simulink model "Lab4_6_StudentVersion"  (R2025a)
settings: Solver=VariableStepAuto  StartTime=0.0  StopTime=30  FixedStep=5e-5  MaxStep=1e-4  RelTol=1e-6
values from neighbouring files (symbols this model uses):
  Ke1 = 10    [ParametersLAb4_6_StudentVersion.m]
  Ke2 = 10    [ParametersLAb4_6_StudentVersion.m]
  Ki = 4.5e-4    (= 0.00045)    [ParametersLAb4_6_StudentVersion.m]
  Ksi = 1    [ParametersLAb4_6_StudentVersion.m]
  m1 = delta_w/P1_rated    (= 0.00333333333333)    [ParametersLAb4_6_StudentVersion.m]
  m2 = delta_w/P2_rated    (= 0.0025)    [ParametersLAb4_6_StudentVersion.m]
  n1 = delta_V/Q1_rated    (= 0.000666666666667)    [ParametersLAb4_6_StudentVersion.m]
  n2 = delta_V/Q2_rated    (= 0.00133333333333)    [ParametersLAb4_6_StudentVersion.m]
  P1_rated = 3000    [ParametersLAb4_6_StudentVersion.m]
  P2_rated = 4000    [ParametersLAb4_6_StudentVersion.m]
  Q1_rated = 1500    [ParametersLAb4_6_StudentVersion.m]
  Q2_rated = 1500/2    (= 750)    [ParametersLAb4_6_StudentVersion.m]
  Rf = 0.1    [ParametersLAb4_6_StudentVersion.m]
  T32 = sqrt(2/3)*[   1      0 ... (first row only)    [ParametersLAb4_6_StudentVersion.m]
  Tf = 0.1    [ParametersLAb4_6_StudentVersion.m]
  V1_rated = 110    [ParametersLAb4_6_StudentVersion.m]
  V2_rated = 110    [ParametersLAb4_6_StudentVersion.m]
  w1_rated = 2*pi*f1_rated    (= 376.991118431)    [ParametersLAb4_6_StudentVersion.m]
  w2_rated = 2*pi*f2_rated    (= 376.991118431)    [ParametersLAb4_6_StudentVersion.m]
  wne = 500    [ParametersLAb4_6_StudentVersion.m]
libraries: fl_lib x33, nesl_utility x31, ee_lib x22
(part 2 of 2)

== system Lab4_6_StudentVersion/Subsystem8 ==
  PS-Simulink Converter : nesl_utility/PS-Simulink Converter  PhysicalDomain=network_engine_domain  SubClassName=ps_output  LeftPortType=input  RightPortType=output  PseudoPeriodic=off  Frequencies=[]  VectorFormat=inherit  Unit=inherit  AffineConversion=off
  Voltage Sensor : fl_lib/Electrical/Electrical Sensors/Voltage Sensor
  + : PMIOPort  Side=Right
  - : PMIOPort  Port=2  Side=Right
  V : Outport
  wires:
  PS-Simulink Converter/1 -> V/1
  connections:
  Voltage Sensor/RConn2 -- -/RConn1
  PS-Simulink Converter/LConn1 -- Voltage Sensor/RConn1
  Voltage Sensor/LConn1 -- +/RConn1

== system Lab4_6_StudentVersion/Subsystem9 ==
  PS-Simulink Converter : nesl_utility/PS-Simulink Converter  PhysicalDomain=network_engine_domain  SubClassName=ps_output  LeftPortType=input  RightPortType=output  PseudoPeriodic=off  Frequencies=[]  VectorFormat=inherit  Unit=inherit  AffineConversion=off
  Voltage Sensor : fl_lib/Electrical/Electrical Sensors/Voltage Sensor
  + : PMIOPort  Side=Right
  - : PMIOPort  Port=2  Side=Right
  V : Outport
  wires:
  PS-Simulink Converter/1 -> V/1
  connections:
  Voltage Sensor/LConn1 -- +/RConn1
  PS-Simulink Converter/LConn1 -- Voltage Sensor/RConn1
  Voltage Sensor/RConn2 -- -/RConn1

== system Lab4_6_StudentVersion/CPL/0dq-abc ==
  d : Inport
  q : Inport  Port=2
  theta : Inport  Port=3
  Fcn1 : Fcn  Expr=sqrt(2/3)*(u[1]/sqrt(2)+u[2]*cos(u[4]-2*pi/3)-u[3]*sin(u[4]-2*pi/3))
  Fcn2 : Fcn  Expr=sqrt(2/3)*(u[1]/sqrt(2)+u[2]*cos(u[4]-4*pi/3)-u[3]*sin(u[4]-4*pi/3))
  Fcn3 : Fcn  Expr=sqrt(2/3)*(u[1]/sqrt(2)+u[2]*cos(u[4])-u[3]*sin(u[4]))
  Mux2 : Mux
  a : Outport  InitialOutput=0
  b : Outport  Port=2  InitialOutput=0
  c : Outport  Port=3  InitialOutput=0
  wires:
  Mux2/1 -> Fcn1/1, Fcn2/1, Fcn3/1
  theta/1 -> Mux2/4
  d/1 -> Mux2/2
  q/1 -> Mux2/3
  Fcn3/1 -> a/1
  Fcn1/1 -> b/1
  Fcn2/1 -> c/1

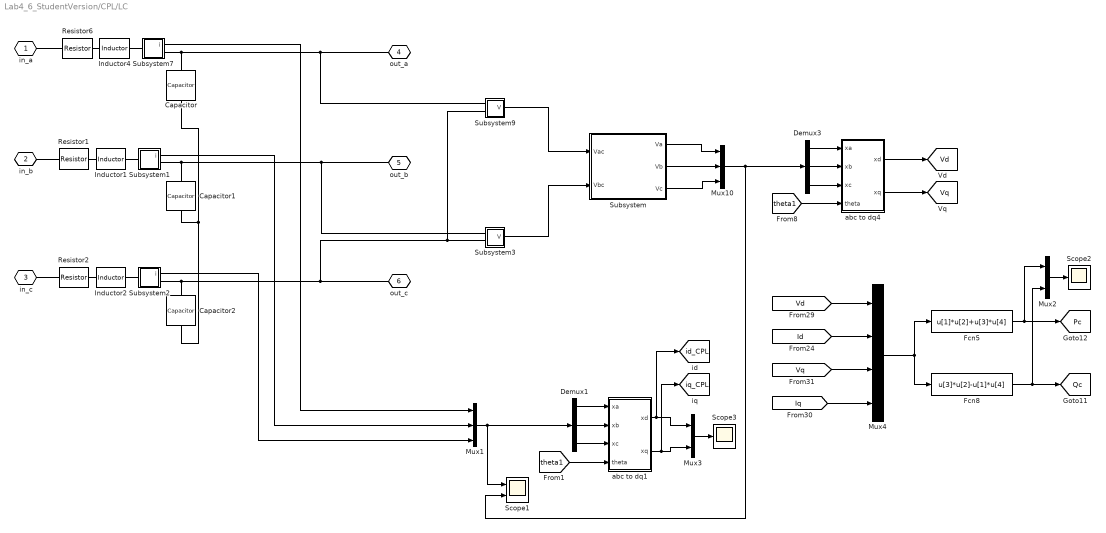
== system Lab4_6_StudentVersion/CPL/LC ==
  Capacitor : fl_lib/Electrical/Electrical Elements/Capacitor  c=Cf F  r=1e-6 Ohm  g=0 1/Ohm  i_specify=off  i_priority=None  i=0 A  i_nominal_specify=off  i_nominal_value=1  i_nominal_unit=A  v_specify=on  v_priority=None  v=V1_rated V  v_nominal_specify=off  v_nominal_value=1  v_nominal_unit=V  vc_specify=on  vc_priority=High  vc=V1_rated V  vc_nominal_specify=off  vc_nominal_value=1  vc_nominal_unit=V
  Capacitor1 : fl_lib/Electrical/Electrical Elements/Capacitor  c=Cf F  r=1e-6 Ohm  g=0 1/Ohm  i_specify=off  i_priority=None  i=0 A  i_nominal_specify=off  i_nominal_value=1  i_nominal_unit=A  v_specify=on  v_priority=None  v=V1_rated*sin(-2*pi/3) V  v_nominal_specify=off  v_nominal_value=1  v_nominal_unit=V  vc_specify=on  vc_priority=High  vc=V1_rated*sin(-2*pi/3) V  vc_nominal_specify=off  vc_nominal_value=1  vc_nominal_unit=V
  Capacitor2 : fl_lib/Electrical/Electrical Elements/Capacitor  c=Cf F  r=1e-6 Ohm  g=0 1/Ohm  i_specify=off  i_priority=None  i=0 A  i_nominal_specify=off  i_nominal_value=1  i_nominal_unit=A  v_specify=on  v_priority=None  v=V1_rated*sin(2*pi/3) V  v_nominal_specify=off  v_nominal_value=1  v_nominal_unit=V  vc_specify=on  vc_priority=High  vc=V1_rated*sin(2*pi/3) V  vc_nominal_specify=off  vc_nominal_value=1  vc_nominal_unit=V
  Demux1 : Demux  Outputs=3
  Demux3 : Demux  Outputs=3
  Fcn5 : Fcn  Expr=u[1]*u[2]+u[3]*u[4]
  Fcn8 : Fcn  Expr=u[3]*u[2]-u[1]*u[4]
  Inductor1 : ee_lib/Passive/Inductor  l=Lf H  enable_L_tol=ee.enum.toleranceApplication.none  L_tol=20  tol_distribution=ee.enum.toleranceDistribution.uniform  nSigma=4  r=0 Ohm  g=1e-9 1/Ohm  enable_operating_limits=ee.enum.enable.no  operating_limit_action=ee.enum.passive.reportOpLim.warn  max_working_current=1 A  power_rating=1 W  i_L_specify=on  i_L_priority=High  i_L=3 A  i_L_nominal_specify=off  i_L_nominal_value=1  i_L_nominal_unit=A
  Inductor2 : ee_lib/Passive/Inductor  l=Lf H  enable_L_tol=ee.enum.toleranceApplication.none  L_tol=20  tol_distribution=ee.enum.toleranceDistribution.uniform  nSigma=4  r=0 Ohm  g=1e-9 1/Ohm  enable_operating_limits=ee.enum.enable.no  operating_limit_action=ee.enum.passive.reportOpLim.warn  max_working_current=1 A  power_rating=1 W  i_L_specify=on  i_L_priority=High  i_L=3 A  i_L_nominal_specify=off  i_L_nominal_value=1  i_L_nominal_unit=A
  Inductor4 : ee_lib/Passive/Inductor  l=Lf H  enable_L_tol=ee.enum.toleranceApplication.none  L_tol=20  tol_distribution=ee.enum.toleranceDistribution.uniform  nSigma=4  r=0 Ohm  g=1e-9 1/Ohm  enable_operating_limits=ee.enum.enable.no  operating_limit_action=ee.enum.passive.reportOpLim.warn  max_working_current=1 A  power_rating=1 W  i_L_specify=on  i_L_priority=High  i_L=3 A  i_L_nominal_specify=off  i_L_nominal_value=1  i_L_nominal_unit=A
  Mux1 : Mux  Inputs=3
  Mux10 : Mux  Inputs=3
  Mux2 : Mux  Inputs=2
  Mux3 : Mux  Inputs=2
  Mux4 : Mux
  Resistor1 : ee_lib/Passive/Resistor  R=Rf Ohm  enable_R_tol=ee.enum.toleranceApplication.none  R_tol=5  tol_distribution=ee.enum.toleranceDistribution.uniform  nSigma=4  enable_operating_limits=ee.enum.enable.no  operating_limit_action=ee.enum.passive.reportOpLim.warn  power_rating=1 W  max_working_voltage=100 V  noise_mode=ee.enum.sources.noise.Disabled  Tdevice=25 degC  sample_time=1e-3 s  repeatability=ee.enum.ic.repeatability.notRepeatable  user_seed=0  auto_seed=3402504572  power_derating_T1=70 degC  power_derating_T2=155 degC  operating_temperature_range_vec=[-50, 150] degC  alpha=3.93e-3 1/K  Tmeas=25 degC  thermal_mass=100 J/K  temperature_specify=off  temperature_priority=High  temperature=298.15 K  temperature_nominal_specify=off  temperature_nominal_value=1  temperature_nominal_unit=K
  Resistor2 : ee_lib/Passive/Resistor  R=Rf Ohm  enable_R_tol=ee.enum.toleranceApplication.none  R_tol=5  tol_distribution=ee.enum.toleranceDistribution.uniform  nSigma=4  enable_operating_limits=ee.enum.enable.no  operating_limit_action=ee.enum.passive.reportOpLim.warn  power_rating=1 W  max_working_voltage=100 V  noise_mode=ee.enum.sources.noise.Disabled  Tdevice=25 degC  sample_time=1e-3 s  repeatability=ee.enum.ic.repeatability.notRepeatable  user_seed=0  auto_seed=4120988592  power_derating_T1=70 degC  power_derating_T2=155 degC  operating_temperature_range_vec=[-50, 150] degC  alpha=3.93e-3 1/K  Tmeas=25 degC  thermal_mass=100 J/K  temperature_specify=off  temperature_priority=High  temperature=298.15 K  temperature_nominal_specify=off  temperature_nominal_value=1  temperature_nominal_unit=K
  Resistor6 : ee_lib/Passive/Resistor  R=Rf Ohm  enable_R_tol=ee.enum.toleranceApplication.none  R_tol=5  tol_distribution=ee.enum.toleranceDistribution.uniform  nSigma=4  enable_operating_limits=ee.enum.enable.no  operating_limit_action=ee.enum.passive.reportOpLim.warn  power_rating=1 W  max_working_voltage=100 V  noise_mode=ee.enum.sources.noise.Disabled  Tdevice=25 degC  sample_time=1e-3 s  repeatability=ee.enum.ic.repeatability.notRepeatable  user_seed=0  auto_seed=3933054132  power_derating_T1=70 degC  power_derating_T2=155 degC  operating_temperature_range_vec=[-50, 150] degC  alpha=3.93e-3 1/K  Tmeas=25 degC  thermal_mass=100 J/K  temperature_specify=off  temperature_priority=High  temperature=298.15 K  temperature_nominal_specify=off  temperature_nominal_value=1  temperature_nominal_unit=K
  Scope1 : Scope  NumInputPorts=2
      settings: TimeSpan=0.06097832817337462  ActiveDisplayYMinimum=-7.7647058823528994  ActiveDisplayYMaximum=6.8235294117647394  DataLoggingVariableName=ScopeData5
  Scope2 : Scope
      settings: TimeSpan=0.02490302560124127  ActiveDisplayYMinimum=-200  ActiveDisplayYMaximum=225  DataLoggingVariableName=ScopeData25
  Scope3 : Scope
      settings: TimeSpan=0.02490302560124127  ActiveDisplayYMinimum=-200  ActiveDisplayYMaximum=225  DataLoggingVariableName=ScopeData31
  Subsystem : Subsystem
  Subsystem1 : Subsystem
  Subsystem2 : Subsystem
  Subsystem3 : Subsystem
      settings: PortSchema="{\"entries\":[{\"content\":{\"sides\":[{\"content\":{\"connectorIds\":[\"Out1\"]},\"type\":\"ConnectorPlacement.EquallySpacedRectSide\",\"uuid\":\"f9dae77b-82ec-46c0-8ec7-07c4c343cd61\"},{\"content\":{\"connectorIds\":[\"RConn1\",\"RConn2\"],\"side\":\"RIGHT\"},\"type\":\"ConnectorPlacement.EquallySpacedRectSide\",\"uuid\":\"c868f1e8-59aa-45a3-abdf-5b79dca1cbd6\"},{\"content\":{\"side\":\"TOP\"},\"type\":\"ConnectorPlacement.EquallySpacedRectSide\",\"uuid\":\"1fe3fd4f-ec18-4909-aef2-795910f5eee8\"},{\"content\":{\"side\":\"BOTTOM\"},\"type\":\"ConnectorPlacement.EquallySpacedRectSide\",\"uuid\":\"67a88f15-4497-4048-9449-885deab38afe\"}]},\"type\":\"ConnectorPlacement.EquallySpacedConnector\",\"uuid\":\"b65f0ac3-40cf-4bf8-a5c1-5ed6a13721a4\"}],\"packageUris\":[\"http://schema.mathworks.com/mf0/Connector/R2020b\"],\"version\":\"1.0\"}"
  Subsystem7 : Subsystem
  Subsystem9 : Subsystem
      settings: PortSchema="{\"entries\":[{\"content\":{\"sides\":[{\"content\":{\"connectorIds\":[\"Out1\"]},\"type\":\"ConnectorPlacement.EquallySpacedRectSide\",\"uuid\":\"f9dae77b-82ec-46c0-8ec7-07c4c343cd61\"},{\"content\":{\"connectorIds\":[\"RConn1\",\"RConn2\"],\"side\":\"RIGHT\"},\"type\":\"ConnectorPlacement.EquallySpacedRectSide\",\"uuid\":\"c868f1e8-59aa-45a3-abdf-5b79dca1cbd6\"},{\"content\":{\"side\":\"TOP\"},\"type\":\"ConnectorPlacement.EquallySpacedRectSide\",\"uuid\":\"1fe3fd4f-ec18-4909-aef2-795910f5eee8\"},{\"content\":{\"side\":\"BOTTOM\"},\"type\":\"ConnectorPlacement.EquallySpacedRectSide\",\"uuid\":\"67a88f15-4497-4048-9449-885deab38afe\"}]},\"type\":\"ConnectorPlacement.EquallySpacedConnector\",\"uuid\":\"b65f0ac3-40cf-4bf8-a5c1-5ed6a13721a4\"}],\"packageUris\":[\"http://schema.mathworks.com/mf0/Connector/R2020b\"],\"version\":\"1.0\"}"
  abc to dq1 : Subsystem
  abc to dq4 : Subsystem
  in_a : PMIOPort  Tag=PMCPort  Side=Right
  in_b : PMIOPort  Tag=PMCPort  Port=2  Side=Right
  in_c : PMIOPort  Tag=PMCPort  Port=3  Side=Right
  out_a : PMIOPort  Tag=PMCPort  Port=4  Side=Left
  out_b : PMIOPort  Tag=PMCPort  Port=5  Side=Left
  out_c : PMIOPort  Tag=PMCPort  Port=6  Side=Left
  tag scope: Pc=global, Qc=global, Vd=global, Vq=global, id_CPL=global, iq_CPL=global
  wires:
  Mux10/1 -> Demux3/1, Scope1/2
  Subsystem/3(Vc) -> Mux10/3
  Subsystem/2(Vb) -> Mux10/2
  Subsystem/1(Va) -> Mux10/1
  Subsystem7/1(i) -> Mux1/1
  Subsystem1/1(i) -> Mux1/2
  Subsystem2/1(i) -> Mux1/3
  Demux3/1 -> abc to dq4/1(xa)
  Demux3/2 -> abc to dq4/2(xb)
  Demux3/3 -> abc to dq4/3(xc)
  abc to dq4/1(xd) -> [Vd]
  abc to dq4/2(xq) -> [Vq]
  [theta1] -> abc to dq4/4(theta)
  Subsystem9/1(V) -> Subsystem/1(Vac)
  Subsystem3/1(V) -> Subsystem/2(Vbc)
  Mux4/1 -> Fcn8/1, Fcn5/1
  [Id] -> Mux4/2
  [Iq] -> Mux4/4
  [Vd] -> Mux4/1
  [Vq] -> Mux4/3
  Fcn5/1 -> Mux2/1, [Pc]
  Fcn8/1 -> Mux2/2, [Qc]
  Mux2/1 -> Scope2/1
  Mux1/1 -> Scope1/1, Demux1/1
  Demux1/1 -> abc to dq1/1(xa)
  Demux1/2 -> abc to dq1/2(xb)
  Demux1/3 -> abc to dq1/3(xc)
  abc to dq1/1(xd) -> Mux3/1, [id_CPL]
  abc to dq1/2(xq) -> Mux3/2, [iq_CPL]
  [theta1] -> abc to dq1/4(theta)
  Mux3/1 -> Scope3/1
  connections:
  Subsystem3/RConn1 -- out_b/RConn1 -- Subsystem1/RConn1 -- Capacitor1/LConn1
  Subsystem9/RConn1 -- out_a/RConn1 -- Subsystem7/RConn1 -- Capacitor/LConn1
  out_c/RConn1 -- Subsystem2/RConn1 -- Capacitor2/LConn1 -- Subsystem9/RConn2 -- Subsystem3/RConn2
  Inductor4/LConn1 -- Resistor6/RConn1
  Resistor6/LConn1 -- in_a/RConn1
  Inductor4/RConn1 -- Subsystem7/LConn1
  Inductor1/LConn1 -- Resistor1/RConn1
  Inductor1/RConn1 -- Subsystem1/LConn1
  in_b/RConn1 -- Resistor1/LConn1
  Inductor2/LConn1 -- Resistor2/RConn1
  Inductor2/RConn1 -- Subsystem2/LConn1
  in_c/RConn1 -- Resistor2/LConn1
  Capacitor/RConn1 -- Capacitor1/RConn1 -- Capacitor2/RConn1

== system Lab4_6_StudentVersion/Constant Current Load/0dq-abc ==
  d : Inport
  q : Inport  Port=2
  theta : Inport  Port=3
  Fcn1 : Fcn  Expr=sqrt(2/3)*(u[1]/sqrt(2)+u[2]*cos(u[4]-2*pi/3)-u[3]*sin(u[4]-2*pi/3))
  Fcn2 : Fcn  Expr=sqrt(2/3)*(u[1]/sqrt(2)+u[2]*cos(u[4]-4*pi/3)-u[3]*sin(u[4]-4*pi/3))
  Fcn3 : Fcn  Expr=sqrt(2/3)*(u[1]/sqrt(2)+u[2]*cos(u[4])-u[3]*sin(u[4]))
  Mux2 : Mux
  a : Outport  InitialOutput=0
  b : Outport  Port=2  InitialOutput=0
  c : Outport  Port=3  InitialOutput=0
  wires:
  Mux2/1 -> Fcn1/1, Fcn2/1, Fcn3/1
  theta/1 -> Mux2/4
  d/1 -> Mux2/2
  q/1 -> Mux2/3
  Fcn3/1 -> a/1
  Fcn1/1 -> b/1
  Fcn2/1 -> c/1

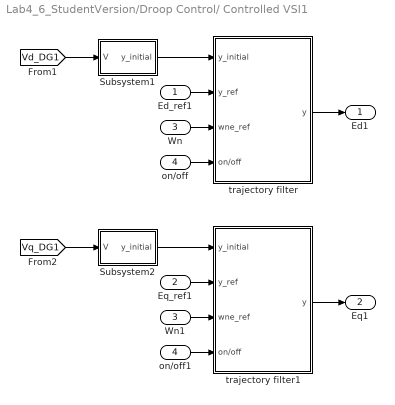
== system Lab4_6_StudentVersion/Droop Control/ Controlled VSI1 ==
  Ed_ref1 : Inport
  Eq_ref1 : Inport  Port=2
  Wn : Inport  Port=3
  on/off : Inport  Port=4
  Subsystem1 : Subsystem
  Subsystem2 : Subsystem
  Wn1 : InportShadow  Port=3
  on/off1 : InportShadow  Port=4
  trajectory filter : Subsystem
  trajectory filter1 : Subsystem
  Ed1 : Outport
  Eq1 : Outport  Port=2
  wires:
  Ed_ref1/1 -> trajectory filter/2(y_ref)
  trajectory filter/1(y) -> Ed1/1
  Eq_ref1/1 -> trajectory filter1/2(y_ref)
  Wn/1 -> trajectory filter/3(wne_ref)
  Subsystem1/1(y_initial) -> trajectory filter/1(y_initial)
  [Vd_DG1] -> Subsystem1/1(V)
  [Vq_DG1] -> Subsystem2/1(V)
  Subsystem2/1(y_initial) -> trajectory filter1/1(y_initial)
  trajectory filter1/1(y) -> Eq1/1
  on/off/1 -> trajectory filter/4(on/off)
  on/off1/1 -> trajectory filter1/4(on/off)
  Wn1/1 -> trajectory filter1/3(wne_ref)

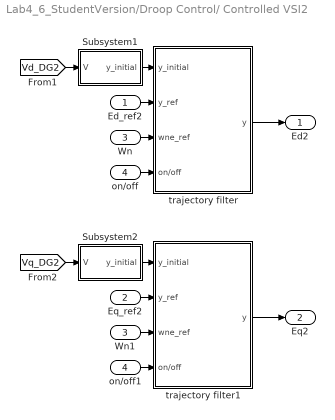
== system Lab4_6_StudentVersion/Droop Control/ Controlled VSI2 ==
  Ed_ref2 : Inport
  Eq_ref2 : Inport  Port=2
  Wn : Inport  Port=3
  on/off : Inport  Port=4
  Subsystem1 : Subsystem
  Subsystem2 : Subsystem
  Wn1 : InportShadow  Port=3
  on/off1 : InportShadow  Port=4
  trajectory filter : Subsystem
  trajectory filter1 : Subsystem
  Ed2 : Outport
  Eq2 : Outport  Port=2
  wires:
  Wn/1 -> trajectory filter/3(wne_ref)
  Subsystem1/1(y_initial) -> trajectory filter/1(y_initial)
  trajectory filter1/1(y) -> Eq2/1
  [Vd_DG2] -> Subsystem1/1(V)
  trajectory filter/1(y) -> Ed2/1
  on/off1/1 -> trajectory filter1/4(on/off)
  Ed_ref2/1 -> trajectory filter/2(y_ref)
  [Vq_DG2] -> Subsystem2/1(V)
  Subsystem2/1(y_initial) -> trajectory filter1/1(y_initial)
  Eq_ref2/1 -> trajectory filter1/2(y_ref)
  on/off/1 -> trajectory filter/4(on/off)
  Wn1/1 -> trajectory filter1/3(wne_ref)

== system Lab4_6_StudentVersion/Droop Control/0dq-abc ==
  d : Inport
  q : Inport  Port=2
  theta : Inport  Port=3
  Fcn1 : Fcn  Expr=sqrt(2/3)*(u[1]/sqrt(2)+u[2]*cos(u[4]-2*pi/3)-u[3]*sin(u[4]-2*pi/3))
  Fcn2 : Fcn  Expr=sqrt(2/3)*(u[1]/sqrt(2)+u[2]*cos(u[4]-4*pi/3)-u[3]*sin(u[4]-4*pi/3))
  Fcn3 : Fcn  Expr=sqrt(2/3)*(u[1]/sqrt(2)+u[2]*cos(u[4])-u[3]*sin(u[4]))
  Mux2 : Mux
  a : Outport  InitialOutput=0
  b : Outport  Port=2  InitialOutput=0
  c : Outport  Port=3  InitialOutput=0
  wires:
  Mux2/1 -> Fcn1/1, Fcn2/1, Fcn3/1
  theta/1 -> Mux2/4
  d/1 -> Mux2/2
  q/1 -> Mux2/3
  Fcn3/1 -> a/1
  Fcn1/1 -> b/1
  Fcn2/1 -> c/1

== system Lab4_6_StudentVersion/Droop Control/0dq-abc1 ==
  d : Inport
  q : Inport  Port=2
  theta : Inport  Port=3
  Fcn1 : Fcn  Expr=sqrt(2/3)*(u[1]/sqrt(2)+u[2]*cos(u[4]-2*pi/3)-u[3]*sin(u[4]-2*pi/3))
  Fcn2 : Fcn  Expr=sqrt(2/3)*(u[1]/sqrt(2)+u[2]*cos(u[4]-4*pi/3)-u[3]*sin(u[4]-4*pi/3))
  Fcn3 : Fcn  Expr=sqrt(2/3)*(u[1]/sqrt(2)+u[2]*cos(u[4])-u[3]*sin(u[4]))
  Mux2 : Mux
  a : Outport  InitialOutput=0
  b : Outport  Port=2  InitialOutput=0
  c : Outport  Port=3  InitialOutput=0
  wires:
  Fcn2/1 -> c/1
  Fcn1/1 -> b/1
  Fcn3/1 -> a/1
  q/1 -> Mux2/3
  d/1 -> Mux2/2
  theta/1 -> Mux2/4
  Mux2/1 -> Fcn3/1, Fcn2/1, Fcn1/1

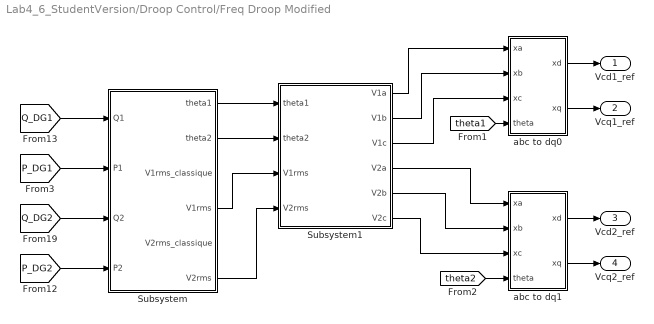
== system Lab4_6_StudentVersion/Droop Control/Freq Droop Modified ==
  Subsystem : Subsystem
  Subsystem1 : Subsystem
  abc to dq0 : Subsystem
  abc to dq1 : Subsystem
  Vcd1_ref : Outport
  Vcq1_ref : Outport  Port=2
  Vcd2_ref : Outport  Port=3
  Vcq2_ref : Outport  Port=4
  wires:
  [Q_DG2] -> Subsystem/3(Q2)
  [Q_DG1] -> Subsystem/1(Q1)
  [P_DG2] -> Subsystem/4(P2)
  [P_DG1] -> Subsystem/2(P1)
  Subsystem1/1(V1a) -> abc to dq0/1(xa)
  Subsystem1/2(V1b) -> abc to dq0/2(xb)
  Subsystem1/3(V1c) -> abc to dq0/3(xc)
  Subsystem1/4(V2a) -> abc to dq1/1(xa)
  Subsystem1/5(V2b) -> abc to dq1/2(xb)
  Subsystem1/6(V2c) -> abc to dq1/3(xc)
  [theta1] -> abc to dq0/4(theta)
  [theta2] -> abc to dq1/4(theta)
  Subsystem/1(theta1) -> Subsystem1/1(theta1)
  Subsystem/2(theta2) -> Subsystem1/2(theta2)
  abc to dq1/1(xd) -> Vcd2_ref/1
  abc to dq1/2(xq) -> Vcq2_ref/1
  abc to dq0/1(xd) -> Vcd1_ref/1
  abc to dq0/2(xq) -> Vcq1_ref/1
  Subsystem/4(V1rms) -> Subsystem1/3(V1rms)
  Subsystem/6(V2rms) -> Subsystem1/4(V2rms)

== system Lab4_6_StudentVersion/Droop Control/abc to dq4 ==
  xa : Inport
  xb : Inport  Port=2
  xc : Inport  Port=3
  theta : Inport  Port=4
  Fcn : Fcn  Expr=sqrt(2/3)*(u[1]*cos(u[4])+u[2]*cos(u[4]-2*pi/3)+u[3]*cos(u[4]-4*pi/3))
  Fcn1 : Fcn  Expr=sqrt(2/3)*(-u[1]*sin(u[4])-u[2]*sin(u[4]-2*pi/3)-u[3]*sin(u[4]-4*pi/3))
  Fcn2 : Fcn  Expr=sqrt(2/3)*(u[1]+u[2]+u[3])/sqrt(2)
  Mux : Mux
  xd : Outport  VectorParamsAs1DForOutWhenUnconnected=off
  xq : Outport  Port=2  VectorParamsAs1DForOutWhenUnconnected=off
  wires:
  theta/1 -> Mux/4
  xc/1 -> Mux/3
  xb/1 -> Mux/2
  xa/1 -> Mux/1
  Fcn1/1 -> xq/1
  Fcn/1 -> xd/1
  Mux/1 -> Fcn2/1, Fcn/1, Fcn1/1

== system Lab4_6_StudentVersion/Measurements/Subsystem ==
  Vd : Inport
  Vq : Inport  Port=2
  Fcn2 : Fcn  Expr=atan(u(2)/u(1))
  Fcn4 : Fcn  Expr=sqrt(u[1]^2+u[2]^2)
  Gain4 : Gain  Gain=sqrt(1/3)
  Mux6 : Mux  Inputs=2
  Subsystem2 : Subsystem
  Vrms : Outport
  delta : Outport  Port=2
  wires:
  Gain4/1 -> Vrms/1
  Mux6/1 -> Fcn4/1, Fcn2/1
  Subsystem2/1(out) -> Mux6/1
  Fcn4/1 -> Gain4/1
  Vq/1 -> Mux6/2
  Fcn2/1 -> delta/1
  Vd/1 -> Subsystem2/1(V)

== system Lab4_6_StudentVersion/Measurements/Subsystem2 ==
  Vd : Inport
  Vq : Inport  Port=2
  Fcn2 : Fcn  Expr=atan(u(2)/u(1))
  Fcn4 : Fcn  Expr=sqrt(u[1]^2+u[2]^2)
  Gain4 : Gain  Gain=sqrt(1/3)
  Mux6 : Mux  Inputs=2
  Subsystem2 : Subsystem
  Vrms : Outport
  delta : Outport  Port=2
  wires:
  Vd/1 -> Subsystem2/1(V)
  Fcn2/1 -> delta/1
  Vq/1 -> Mux6/2
  Fcn4/1 -> Gain4/1
  Subsystem2/1(out) -> Mux6/1
  Mux6/1 -> Fcn2/1, Fcn4/1
  Gain4/1 -> Vrms/1

== system Lab4_6_StudentVersion/Measurements/abc to dq0 ==
  xa : Inport
  xb : Inport  Port=2
  xc : Inport  Port=3
  theta : Inport  Port=4
  Fcn : Fcn  Expr=sqrt(2/3)*(u[1]*cos(u[4])+u[2]*cos(u[4]-2*pi/3)+u[3]*cos(u[4]-4*pi/3))
  Fcn1 : Fcn  Expr=sqrt(2/3)*(-u[1]*sin(u[4])-u[2]*sin(u[4]-2*pi/3)-u[3]*sin(u[4]-4*pi/3))
  Fcn2 : Fcn  Expr=sqrt(2/3)*(u[1]+u[2]+u[3])/sqrt(2)
  Mux : Mux
  xd : Outport
  xq : Outport  Port=2
  wires:
  Mux/1 -> Fcn1/1, Fcn/1, Fcn2/1
  Fcn/1 -> xd/1
  Fcn1/1 -> xq/1
  xa/1 -> Mux/1
  xb/1 -> Mux/2
  xc/1 -> Mux/3
  theta/1 -> Mux/4

== system Lab4_6_StudentVersion/Measurements/abc to dq1 ==
  xa : Inport
  xb : Inport  Port=2
  xc : Inport  Port=3
  theta : Inport  Port=4
  Fcn : Fcn  Expr=sqrt(2/3)*(u[1]*cos(u[4])+u[2]*cos(u[4]-2*pi/3)+u[3]*cos(u[4]-4*pi/3))
  Fcn1 : Fcn  Expr=sqrt(2/3)*(-u[1]*sin(u[4])-u[2]*sin(u[4]-2*pi/3)-u[3]*sin(u[4]-4*pi/3))
  Fcn2 : Fcn  Expr=sqrt(2/3)*(u[1]+u[2]+u[3])/sqrt(2)
  Mux : Mux
  xd : Outport
  xq : Outport  Port=2
  wires:
  theta/1 -> Mux/4
  xc/1 -> Mux/3
  xb/1 -> Mux/2
  xa/1 -> Mux/1
  Fcn1/1 -> xq/1
  Fcn/1 -> xd/1
  Mux/1 -> Fcn2/1, Fcn/1, Fcn1/1

== system Lab4_6_StudentVersion/Measurements/abc to dq2 ==
  xa : Inport
  xb : Inport  Port=2
  xc : Inport  Port=3
  theta : Inport  Port=4
  Fcn : Fcn  Expr=sqrt(2/3)*(u[1]*cos(u[4])+u[2]*cos(u[4]-2*pi/3)+u[3]*cos(u[4]-4*pi/3))
  Fcn1 : Fcn  Expr=sqrt(2/3)*(-u[1]*sin(u[4])-u[2]*sin(u[4]-2*pi/3)-u[3]*sin(u[4]-4*pi/3))
  Fcn2 : Fcn  Expr=sqrt(2/3)*(u[1]+u[2]+u[3])/sqrt(2)
  Mux : Mux
  xd : Outport
  xq : Outport  Port=2
  wires:
  theta/1 -> Mux/4
  xc/1 -> Mux/3
  xb/1 -> Mux/2
  xa/1 -> Mux/1
  Fcn1/1 -> xq/1
  Fcn/1 -> xd/1
  Mux/1 -> Fcn2/1, Fcn/1, Fcn1/1

== system Lab4_6_StudentVersion/Measurements/abc to dq3 ==
  xa : Inport
  xb : Inport  Port=2
  xc : Inport  Port=3
  theta : Inport  Port=4
  Fcn : Fcn  Expr=sqrt(2/3)*(u[1]*cos(u[4])+u[2]*cos(u[4]-2*pi/3)+u[3]*cos(u[4]-4*pi/3))
  Fcn1 : Fcn  Expr=sqrt(2/3)*(-u[1]*sin(u[4])-u[2]*sin(u[4]-2*pi/3)-u[3]*sin(u[4]-4*pi/3))
  Fcn2 : Fcn  Expr=sqrt(2/3)*(u[1]+u[2]+u[3])/sqrt(2)
  Mux : Mux
  xd : Outport
  xq : Outport  Port=2
  wires:
  Mux/1 -> Fcn1/1, Fcn/1, Fcn2/1
  Fcn/1 -> xd/1
  Fcn1/1 -> xq/1
  xa/1 -> Mux/1
  xb/1 -> Mux/2
  xc/1 -> Mux/3
  theta/1 -> Mux/4

== system Lab4_6_StudentVersion/Measurements/abc to dq4 ==
  xa : Inport
  xb : Inport  Port=2
  xc : Inport  Port=3
  theta : Inport  Port=4
  Fcn : Fcn  Expr=sqrt(2/3)*(u[1]*cos(u[4])+u[2]*cos(u[4]-2*pi/3)+u[3]*cos(u[4]-4*pi/3))
  Fcn1 : Fcn  Expr=sqrt(2/3)*(-u[1]*sin(u[4])-u[2]*sin(u[4]-2*pi/3)-u[3]*sin(u[4]-4*pi/3))
  Fcn2 : Fcn  Expr=sqrt(2/3)*(u[1]+u[2]+u[3])/sqrt(2)
  Mux : Mux
  xd : Outport  VectorParamsAs1DForOutWhenUnconnected=off
  xq : Outport  Port=2  VectorParamsAs1DForOutWhenUnconnected=off
  wires:
  theta/1 -> Mux/4
  xc/1 -> Mux/3
  xb/1 -> Mux/2
  xa/1 -> Mux/1
  Fcn1/1 -> xq/1
  Fcn/1 -> xd/1
  Mux/1 -> Fcn2/1, Fcn/1, Fcn1/1

== system Lab4_6_StudentVersion/Measurements/abc to dq5 ==
  xa : Inport
  xb : Inport  Port=2
  xc : Inport  Port=3
  theta : Inport  Port=4
  Fcn : Fcn  Expr=sqrt(2/3)*(u[1]*cos(u[4])+u[2]*cos(u[4]-2*pi/3)+u[3]*cos(u[4]-4*pi/3))
  Fcn1 : Fcn  Expr=sqrt(2/3)*(-u[1]*sin(u[4])-u[2]*sin(u[4]-2*pi/3)-u[3]*sin(u[4]-4*pi/3))
  Fcn2 : Fcn  Expr=sqrt(2/3)*(u[1]+u[2]+u[3])/sqrt(2)
  Mux : Mux
  xd : Outport  VectorParamsAs1DForOutWhenUnconnected=off
  xq : Outport  Port=2  VectorParamsAs1DForOutWhenUnconnected=off
  wires:
  theta/1 -> Mux/4
  xc/1 -> Mux/3
  xb/1 -> Mux/2
  xa/1 -> Mux/1
  Fcn1/1 -> xq/1
  Fcn/1 -> xd/1
  Mux/1 -> Fcn2/1, Fcn/1, Fcn1/1

== system Lab4_6_StudentVersion/Measurements/abc to dq6 ==
  xa : Inport
  xb : Inport  Port=2
  xc : Inport  Port=3
  theta : Inport  Port=4
  Fcn : Fcn  Expr=sqrt(2/3)*(u[1]*cos(u[4])+u[2]*cos(u[4]-2*pi/3)+u[3]*cos(u[4]-4*pi/3))
  Fcn1 : Fcn  Expr=sqrt(2/3)*(-u[1]*sin(u[4])-u[2]*sin(u[4]-2*pi/3)-u[3]*sin(u[4]-4*pi/3))
  Fcn2 : Fcn  Expr=sqrt(2/3)*(u[1]+u[2]+u[3])/sqrt(2)
  Mux : Mux
  xd : Outport
  xq : Outport  Port=2
  wires:
  theta/1 -> Mux/4
  xc/1 -> Mux/3
  xb/1 -> Mux/2
  xa/1 -> Mux/1
  Fcn1/1 -> xq/1
  Fcn/1 -> xd/1
  Mux/1 -> Fcn2/1, Fcn/1, Fcn1/1

== system Lab4_6_StudentVersion/Measurements/abc to dq7 ==
  xa : Inport
  xb : Inport  Port=2
  xc : Inport  Port=3
  theta : Inport  Port=4
  Fcn : Fcn  Expr=sqrt(2/3)*(u[1]*cos(u[4])+u[2]*cos(u[4]-2*pi/3)+u[3]*cos(u[4]-4*pi/3))
  Fcn1 : Fcn  Expr=sqrt(2/3)*(-u[1]*sin(u[4])-u[2]*sin(u[4]-2*pi/3)-u[3]*sin(u[4]-4*pi/3))
  Fcn2 : Fcn  Expr=sqrt(2/3)*(u[1]+u[2]+u[3])/sqrt(2)
  Mux : Mux
  xd : Outport
  xq : Outport  Port=2
  wires:
  Mux/1 -> Fcn1/1, Fcn/1, Fcn2/1
  Fcn/1 -> xd/1
  Fcn1/1 -> xq/1
  xa/1 -> Mux/1
  xb/1 -> Mux/2
  xc/1 -> Mux/3
  theta/1 -> Mux/4

== system Lab4_6_StudentVersion/CPL/LC/Subsystem ==
  Vac : Inport
  Vbc : Inport  Port=2
  Demux : Demux  Outputs=3
  Gain : Gain  Gain=T32*T32'  Multiplication=Matrix(K*u)
  Mux : Mux  Inputs=3
  Va : Outport
  Vb : Outport  Port=2
  Vc : Outport  Port=3
  wires:
  Demux/3 -> Vc/1
  Demux/2 -> Vb/1
  Demux/1 -> Va/1
  Gain/1 -> Demux/1
  Mux/1 -> Gain/1
  Vbc/1 -> Mux/2
  Vac/1 -> Mux/1

== system Lab4_6_StudentVersion/CPL/LC/Subsystem1 ==
  Current Sensor : fl_lib/Electrical/Electrical Sensors/Current Sensor
  PS-Simulink Converter : nesl_utility/PS-Simulink Converter  PhysicalDomain=network_engine_domain  SubClassName=ps_output  LeftPortType=input  RightPortType=output  PseudoPeriodic=off  Frequencies=[]  VectorFormat=inherit  Unit=inherit  AffineConversion=off
  + : PMIOPort  Side=Left
  - : PMIOPort  Port=2  Side=Right
  i : Outport
  wires:
  PS-Simulink Converter/1 -> i/1
  connections:
  Current Sensor/RConn2 -- -/RConn1
  Current Sensor/LConn1 -- +/RConn1
  PS-Simulink Converter/LConn1 -- Current Sensor/RConn1

== system Lab4_6_StudentVersion/CPL/LC/Subsystem2 ==
  Current Sensor : fl_lib/Electrical/Electrical Sensors/Current Sensor
  PS-Simulink Converter : nesl_utility/PS-Simulink Converter  PhysicalDomain=network_engine_domain  SubClassName=ps_output  LeftPortType=input  RightPortType=output  PseudoPeriodic=off  Frequencies=[]  VectorFormat=inherit  Unit=inherit  AffineConversion=off
  + : PMIOPort  Side=Left
  - : PMIOPort  Port=2  Side=Right
  i : Outport
  wires:
  PS-Simulink Converter/1 -> i/1
  connections:
  Current Sensor/RConn2 -- -/RConn1
  Current Sensor/LConn1 -- +/RConn1
  PS-Simulink Converter/LConn1 -- Current Sensor/RConn1

== system Lab4_6_StudentVersion/CPL/LC/Subsystem3 ==
  PS-Simulink Converter : nesl_utility/PS-Simulink Converter  PhysicalDomain=network_engine_domain  SubClassName=ps_output  LeftPortType=input  RightPortType=output  PseudoPeriodic=off  Frequencies=[]  VectorFormat=inherit  Unit=inherit  AffineConversion=off
  Voltage Sensor : fl_lib/Electrical/Electrical Sensors/Voltage Sensor
  + : PMIOPort  Side=Right
  - : PMIOPort  Port=2  Side=Right
  V : Outport
  wires:
  PS-Simulink Converter/1 -> V/1
  connections:
  Voltage Sensor/RConn2 -- -/RConn1
  PS-Simulink Converter/LConn1 -- Voltage Sensor/RConn1
  Voltage Sensor/LConn1 -- +/RConn1

== system Lab4_6_StudentVersion/CPL/LC/Subsystem7 ==
  Current Sensor : fl_lib/Electrical/Electrical Sensors/Current Sensor
  PS-Simulink Converter : nesl_utility/PS-Simulink Converter  PhysicalDomain=network_engine_domain  SubClassName=ps_output  LeftPortType=input  RightPortType=output  PseudoPeriodic=off  Frequencies=[]  VectorFormat=inherit  Unit=inherit  AffineConversion=off
  + : PMIOPort  Side=Left
  - : PMIOPort  Port=2  Side=Right
  i : Outport
  wires:
  PS-Simulink Converter/1 -> i/1
  connections:
  Current Sensor/RConn2 -- -/RConn1
  Current Sensor/LConn1 -- +/RConn1
  PS-Simulink Converter/LConn1 -- Current Sensor/RConn1

== system Lab4_6_StudentVersion/CPL/LC/Subsystem9 ==
  PS-Simulink Converter : nesl_utility/PS-Simulink Converter  PhysicalDomain=network_engine_domain  SubClassName=ps_output  LeftPortType=input  RightPortType=output  PseudoPeriodic=off  Frequencies=[]  VectorFormat=inherit  Unit=inherit  AffineConversion=off
  Voltage Sensor : fl_lib/Electrical/Electrical Sensors/Voltage Sensor
  + : PMIOPort  Side=Right
  - : PMIOPort  Port=2  Side=Right
  V : Outport
  wires:
  PS-Simulink Converter/1 -> V/1
  connections:
  Voltage Sensor/LConn1 -- +/RConn1
  PS-Simulink Converter/LConn1 -- Voltage Sensor/RConn1
  Voltage Sensor/RConn2 -- -/RConn1

== system Lab4_6_StudentVersion/CPL/LC/abc to dq1 ==
  xa : Inport
  xb : Inport  Port=2
  xc : Inport  Port=3
  theta : Inport  Port=4
  Fcn : Fcn  Expr=sqrt(2/3)*(u[1]*cos(u[4])+u[2]*cos(u[4]-2*pi/3)+u[3]*cos(u[4]-4*pi/3))
  Fcn1 : Fcn  Expr=sqrt(2/3)*(-u[1]*sin(u[4])-u[2]*sin(u[4]-2*pi/3)-u[3]*sin(u[4]-4*pi/3))
  Fcn2 : Fcn  Expr=sqrt(2/3)*(u[1]+u[2]+u[3])/sqrt(2)
  Mux : Mux
  xd : Outport
  xq : Outport  Port=2
  wires:
  Mux/1 -> Fcn1/1, Fcn/1, Fcn2/1
  Fcn/1 -> xd/1
  Fcn1/1 -> xq/1
  xa/1 -> Mux/1
  xb/1 -> Mux/2
  xc/1 -> Mux/3
  theta/1 -> Mux/4

== system Lab4_6_StudentVersion/CPL/LC/abc to dq4 ==
  xa : Inport
  xb : Inport  Port=2
  xc : Inport  Port=3
  theta : Inport  Port=4
  Fcn : Fcn  Expr=sqrt(2/3)*(u[1]*cos(u[4])+u[2]*cos(u[4]-2*pi/3)+u[3]*cos(u[4]-4*pi/3))
  Fcn1 : Fcn  Expr=sqrt(2/3)*(-u[1]*sin(u[4])-u[2]*sin(u[4]-2*pi/3)-u[3]*sin(u[4]-4*pi/3))
  Fcn2 : Fcn  Expr=sqrt(2/3)*(u[1]+u[2]+u[3])/sqrt(2)
  Mux : Mux
  xd : Outport
  xq : Outport  Port=2
  wires:
  theta/1 -> Mux/4
  xc/1 -> Mux/3
  xb/1 -> Mux/2
  xa/1 -> Mux/1
  Fcn1/1 -> xq/1
  Fcn/1 -> xd/1
  Mux/1 -> Fcn2/1, Fcn/1, Fcn1/1

== system Lab4_6_StudentVersion/Droop Control/ Controlled VSI1/Subsystem1 ==
  V : Inport
  Abs : Abs  SaturateOnIntegerOverflow=off
  Constant5 : Constant  Value=1e-7
  Relational Operator : RelationalOperator  OutDataTypeStr=boolean  InputSameDT=off
  Switch : Switch  SaturateOnIntegerOverflow=off  InputSameDT=off
  y_initial : Outport  VectorParamsAs1DForOutWhenUnconnected=off
  wires:
  Switch/1 -> y_initial/1
  Constant5/1 -> Relational Operator/2, Switch/3
  Relational Operator/1 -> Switch/2
  Abs/1 -> Relational Operator/1
  V/1 -> Switch/1, Abs/1

== system Lab4_6_StudentVersion/Droop Control/ Controlled VSI1/Subsystem2 ==
  V : Inport
  Abs : Abs  SaturateOnIntegerOverflow=off
  Constant5 : Constant  Value=1e-7
  Relational Operator : RelationalOperator  OutDataTypeStr=boolean  InputSameDT=off
  Switch : Switch  SaturateOnIntegerOverflow=off  InputSameDT=off
  y_initial : Outport  VectorParamsAs1DForOutWhenUnconnected=off
  wires:
  V/1 -> Abs/1, Switch/1
  Abs/1 -> Relational Operator/1
  Relational Operator/1 -> Switch/2
  Constant5/1 -> Switch/3, Relational Operator/2
  Switch/1 -> y_initial/1

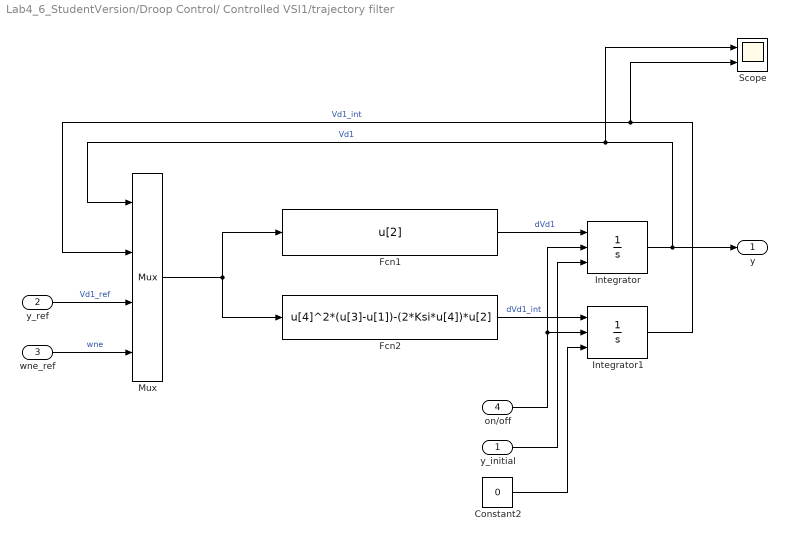
== system Lab4_6_StudentVersion/Droop Control/ Controlled VSI1/trajectory filter ==
  y_initial : Inport
  y_ref : Inport  Port=2
  wne_ref : Inport  Port=3
  on/off : Inport  Port=4
  Constant2 : Constant  Value=0
  Fcn1 : Fcn  Expr=u[2]
  Fcn2 : Fcn  Expr=u[4]^2*(u[3]-u[1])-(2*Ksi*u[4])*u[2]
  Integrator : Integrator  ExternalReset=level  InitialConditionSource=external
  Integrator1 : Integrator  ExternalReset=level  InitialConditionSource=external
  Mux : Mux
  Scope : Scope  NumInputPorts=2
      settings: ActiveDisplayYMinimum=192.6246  ActiveDisplayYMaximum=192.62696  DataLoggingVariableName=ScopeData11
  y : Outport
  wires:
  Mux/1 -> Fcn1/1, Fcn2/1
  Fcn1/1 -> Integrator/1  "dVd1"
  Fcn2/1 -> Integrator1/1  "dVd1_int"
  on/off/1 -> Integrator/2, Integrator1/2
  Constant2/1 -> Integrator1/3
  y_initial/1 -> Integrator/3
  wne_ref/1 -> Mux/4  "wne"
  y_ref/1 -> Mux/3  "Vd1_ref"
  Integrator/1 -> y/1, Scope/1, Mux/1  "Vd1"
  Integrator1/1 -> Scope/2, Mux/2  "Vd1_int"

== system Lab4_6_StudentVersion/Droop Control/ Controlled VSI1/trajectory filter1 ==
  y_initial : Inport
  y_ref : Inport  Port=2
  wne_ref : Inport  Port=3
  on/off : Inport  Port=4
  Constant2 : Constant  Value=0
  Fcn1 : Fcn  Expr=u[2]
  Fcn2 : Fcn  Expr=u[4]^2*(u[3]-u[1])-(2*Ksi*u[4])*u[2]
  Integrator : Integrator  ExternalReset=level  InitialConditionSource=external
  Integrator1 : Integrator  ExternalReset=level  InitialConditionSource=external
  Mux : Mux
  y : Outport
  wires:
  Integrator1/1 -> Mux/2
  Integrator/1 -> Mux/1, y/1
  y_ref/1 -> Mux/3
  wne_ref/1 -> Mux/4
  y_initial/1 -> Integrator/3
  Constant2/1 -> Integrator1/3
  on/off/1 -> Integrator1/2, Integrator/2
  Fcn2/1 -> Integrator1/1
  Fcn1/1 -> Integrator/1
  Mux/1 -> Fcn2/1, Fcn1/1

== system Lab4_6_StudentVersion/Droop Control/ Controlled VSI2/Subsystem1 ==
  V : Inport
  Abs : Abs  SaturateOnIntegerOverflow=off
  Constant5 : Constant  Value=1e-7
  Relational Operator : RelationalOperator  OutDataTypeStr=boolean  InputSameDT=off
  Switch : Switch  SaturateOnIntegerOverflow=off  InputSameDT=off
  y_initial : Outport  VectorParamsAs1DForOutWhenUnconnected=off
  wires:
  Switch/1 -> y_initial/1
  Constant5/1 -> Relational Operator/2, Switch/3
  Relational Operator/1 -> Switch/2
  Abs/1 -> Relational Operator/1
  V/1 -> Switch/1, Abs/1

== system Lab4_6_StudentVersion/Droop Control/ Controlled VSI2/Subsystem2 ==
  V : Inport
  Abs : Abs  SaturateOnIntegerOverflow=off
  Constant5 : Constant  Value=1e-7
  Relational Operator : RelationalOperator  OutDataTypeStr=boolean  InputSameDT=off
  Switch : Switch  SaturateOnIntegerOverflow=off  InputSameDT=off
  y_initial : Outport  VectorParamsAs1DForOutWhenUnconnected=off
  wires:
  V/1 -> Abs/1, Switch/1
  Abs/1 -> Relational Operator/1
  Relational Operator/1 -> Switch/2
  Constant5/1 -> Switch/3, Relational Operator/2
  Switch/1 -> y_initial/1

== system Lab4_6_StudentVersion/Droop Control/ Controlled VSI2/trajectory filter ==
  y_initial : Inport
  y_ref : Inport  Port=2
  wne_ref : Inport  Port=3
  on/off : Inport  Port=4
  Constant2 : Constant  Value=0
  Fcn1 : Fcn  Expr=u[2]
  Fcn2 : Fcn  Expr=u[4]^2*(u[3]-u[1])-(2*Ksi*u[4])*u[2]
  Integrator : Integrator  ExternalReset=level  InitialConditionSource=external
  Integrator1 : Integrator  ExternalReset=level  InitialConditionSource=external
  Mux : Mux
  y : Outport
  wires:
  Mux/1 -> Fcn1/1, Fcn2/1
  Fcn1/1 -> Integrator/1
  Fcn2/1 -> Integrator1/1
  on/off/1 -> Integrator/2, Integrator1/2
  Constant2/1 -> Integrator1/3
  y_initial/1 -> Integrator/3
  wne_ref/1 -> Mux/4
  y_ref/1 -> Mux/3
  Integrator/1 -> y/1, Mux/1
  Integrator1/1 -> Mux/2

== system Lab4_6_StudentVersion/Droop Control/ Controlled VSI2/trajectory filter1 ==
  y_initial : Inport
  y_ref : Inport  Port=2
  wne_ref : Inport  Port=3
  on/off : Inport  Port=4
  Constant2 : Constant  Value=0
  Fcn1 : Fcn  Expr=u[2]
  Fcn2 : Fcn  Expr=u[4]^2*(u[3]-u[1])-(2*Ksi*u[4])*u[2]
  Integrator : Integrator  ExternalReset=level  InitialConditionSource=external
  Integrator1 : Integrator  ExternalReset=level  InitialConditionSource=external
  Mux : Mux
  y : Outport
  wires:
  Integrator1/1 -> Mux/2
  Integrator/1 -> Mux/1, y/1
  y_ref/1 -> Mux/3
  wne_ref/1 -> Mux/4
  y_initial/1 -> Integrator/3
  Constant2/1 -> Integrator1/3
  on/off/1 -> Integrator1/2, Integrator/2
  Fcn2/1 -> Integrator1/1
  Fcn1/1 -> Integrator/1
  Mux/1 -> Fcn2/1, Fcn1/1

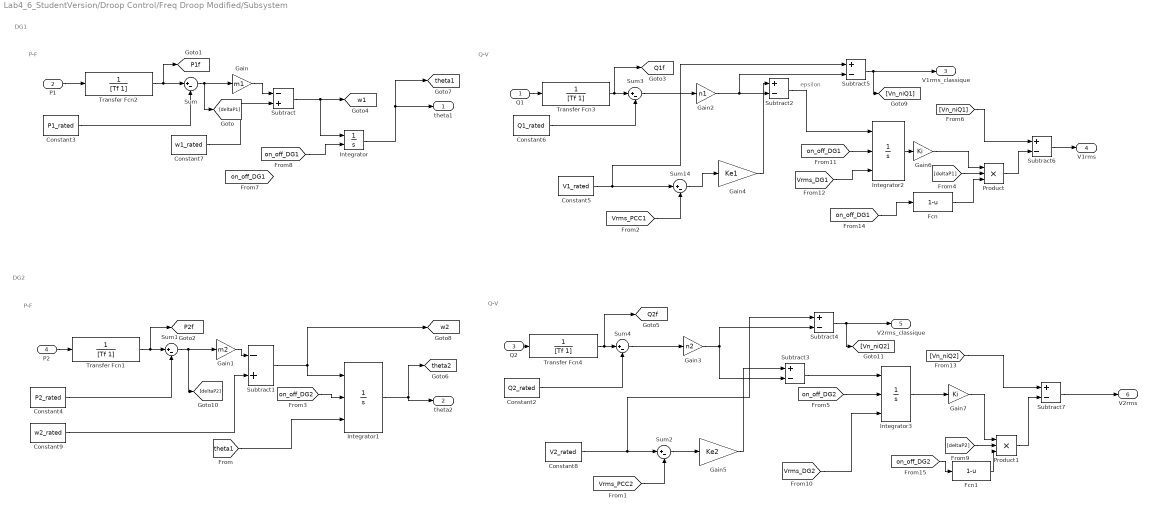
== system Lab4_6_StudentVersion/Droop Control/Freq Droop Modified/Subsystem ==
  note: epsilon
  note: DG1
  note: DG2
  note: P-F
  note: Q-V
  note: P-F
  note: Q-V
  Q1 : Inport
  P1 : Inport  Port=2
  Q2 : Inport  Port=3
  P2 : Inport  Port=4
  Constant2 : Constant  Value=Q2_rated
  Constant3 : Constant  Value=P1_rated
  Constant4 : Constant  Value=P2_rated
  Constant5 : Constant  Value=V1_rated
  Constant6 : Constant  Value=Q1_rated
  Constant7 : Constant  Value=w1_rated
  Constant8 : Constant  Value=V2_rated
  Constant9 : Constant  Value=w2_rated
  Fcn : Fcn  Expr=1-u
  Fcn1 : Fcn  Expr=1-u
  Gain : Gain  Gain=m1
  Gain1 : Gain  Gain=m2
  Gain2 : Gain  Gain=n1
  Gain3 : Gain  Gain=n2
  Gain4 : Gain  Gain=Ke1
  Gain5 : Gain  Gain=Ke2
  Gain6 : Gain  Gain=Ki
  Gain7 : Gain  Gain=Ki
  Integrator : Integrator  ExternalReset=level
  Integrator1 : Integrator  ExternalReset=level  InitialConditionSource=external
  Integrator2 : Integrator  ExternalReset=level  InitialConditionSource=external
  Integrator3 : Integrator  ExternalReset=level  InitialConditionSource=external
  Product : Product  Inputs=3
  Product1 : Product  Inputs=3
  Subtract : Sum  Inputs=-+
  Subtract1 : Sum  Inputs=-+
  Subtract{2..7} (6 alike) : Sum  Inputs=+-
  Sum{,1..4,14} (6 alike) : Sum  Inputs=|+-
  Transfer Fcn{1..4} (4 alike) : TransferFcn  Denominator=[Tf 1]
  theta1 : Outport
  theta2 : Outport  Port=2
  V1rms_classique : Outport  Port=3
  V1rms : Outport  Port=4
  V2rms_classique : Outport  Port=5
  V2rms : Outport  Port=6
  tag scope: P1f=global, P2f=global, Q1f=global, Q2f=global, theta1=global, theta2=global, w1=global, w2=global
  wires:
  P1/1 -> Transfer Fcn2/1
  Transfer Fcn2/1 -> [P1f], Sum/1
  Constant3/1 -> Sum/2
  P2/1 -> Transfer Fcn1/1
  Transfer Fcn1/1 -> [P2f], Sum1/1
  Constant4/1 -> Sum1/2
  Q1/1 -> Transfer Fcn3/1
  Transfer Fcn3/1 -> Sum3/1, [Q1f]
  Constant6/1 -> Sum3/2
  Constant2/1 -> Sum4/2
  Transfer Fcn4/1 -> Sum4/1, [Q2f]
  Q2/1 -> Transfer Fcn4/1
  Constant5/1 -> Subtract5/1, Sum14/1
  [Vrms_PCC1] -> Sum14/2
  Sum14/1 -> Gain4/1
  Sum/1 -> [deltaP1], Gain/1
  Gain/1 -> Subtract/1
  Constant7/1 -> Subtract/2
  Subtract/1 -> Integrator/1, [w1]
  Integrator/1 -> theta1/1, [theta1]
  Sum1/1 -> [deltaP2], Gain1/1
  Gain1/1 -> Subtract1/1
  Constant9/1 -> Subtract1/2
  Subtract1/1 -> [w2], Integrator1/1
  [on_off_DG2] -> Integrator1/2
  Integrator1/1 -> [theta2], theta2/1
  Sum3/1 -> Gain2/1
  Gain2/1 -> Subtract5/2, Subtract2/2
  Subtract2/1 -> Integrator2/1
  Gain4/1 -> Subtract2/1
  Subtract3/1 -> Integrator3/1
  Gain3/1 -> Subtract4/2, Subtract3/2
  Sum4/1 -> Gain3/1
  Gain5/1 -> Subtract3/1
  [on_off_DG1] -> Integrator/2
  Sum2/1 -> Gain5/1
  [Vrms_PCC2] -> Sum2/2
  Constant8/1 -> Subtract4/1, Sum2/1
  [on_off_DG1] -> Integrator2/2
  [on_off_DG2] -> Integrator3/2
  Subtract4/1 -> [Vn_niQ2], V2rms_classique/1
  Subtract5/1 -> [Vn_niQ1], V1rms_classique/1
  [theta1] -> Integrator1/3
  [Vn_niQ1] -> Subtract6/1
  Integrator2/1 -> Gain6/1
  [deltaP1] -> Product/2
  Gain6/1 -> Product/1
  Subtract6/1 -> V1rms/1
  Product/1 -> Subtract6/2
  [Vrms_DG1] -> Integrator2/3
  [deltaP2] -> Product1/2
  Gain7/1 -> Product1/1
  Product1/1 -> Subtract7/2
  Subtract7/1 -> V2rms/1
  [Vn_niQ2] -> Subtract7/1
  Integrator3/1 -> Gain7/1
  [Vrms_DG2] -> Integrator3/3
  Fcn/1 -> Product/3
  [on_off_DG1] -> Fcn/1
  Fcn1/1 -> Product1/3
  [on_off_DG2] -> Fcn1/1

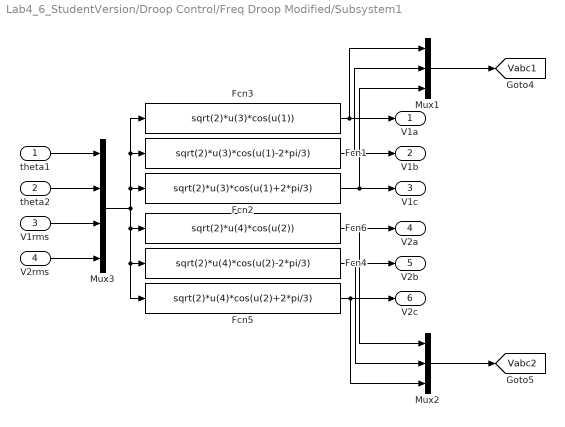
== system Lab4_6_StudentVersion/Droop Control/Freq Droop Modified/Subsystem1 ==
  theta1 : Inport
  theta2 : Inport  Port=2
  V1rms : Inport  Port=3
  V2rms : Inport  Port=4
  Fcn1 : Fcn  Expr=sqrt(2)*u(3)*cos(u(1)-2*pi/3)
  Fcn2 : Fcn  Expr=sqrt(2)*u(3)*cos(u(1)+2*pi/3)
  Fcn3 : Fcn  Expr=sqrt(2)*u(3)*cos(u(1))
  Fcn4 : Fcn  Expr=sqrt(2)*u(4)*cos(u(2)-2*pi/3)
  Fcn5 : Fcn  Expr=sqrt(2)*u(4)*cos(u(2)+2*pi/3)
  Fcn6 : Fcn  Expr=sqrt(2)*u(4)*cos(u(2))
  Mux1 : Mux  Inputs=3
  Mux2 : Mux  Inputs=3
  Mux3 : Mux
  V1a : Outport
  V1b : Outport  Port=2
  V1c : Outport  Port=3
  V2a : Outport  Port=4
  V2b : Outport  Port=5
  V2c : Outport  Port=6
  tag scope: Vabc1=global, Vabc2=global
  wires:
  V2rms/1 -> Mux3/4
  V1rms/1 -> Mux3/3
  theta1/1 -> Mux3/1
  theta2/1 -> Mux3/2
  Mux1/1 -> [Vabc1]
  Mux2/1 -> [Vabc2]
  Mux3/1 -> Fcn5/1, Fcn4/1, Fcn6/1, Fcn3/1, Fcn1/1, Fcn2/1
  Fcn3/1 -> V1a/1, Mux1/1
  Fcn1/1 -> V1b/1, Mux1/2
  Fcn4/1 -> V2b/1, Mux2/2
  Fcn6/1 -> V2a/1, Mux2/1
  Fcn2/1 -> V1c/1, Mux1/3
  Fcn5/1 -> V2c/1, Mux2/3

== system Lab4_6_StudentVersion/Droop Control/Freq Droop Modified/abc to dq0 ==
  xa : Inport
  xb : Inport  Port=2
  xc : Inport  Port=3
  theta : Inport  Port=4
  Fcn : Fcn  Expr=sqrt(2/3)*(u[1]*cos(u[4])+u[2]*cos(u[4]-2*pi/3)+u[3]*cos(u[4]-4*pi/3))
  Fcn1 : Fcn  Expr=sqrt(2/3)*(-u[1]*sin(u[4])-u[2]*sin(u[4]-2*pi/3)-u[3]*sin(u[4]-4*pi/3))
  Fcn2 : Fcn  Expr=sqrt(2/3)*(u[1]+u[2]+u[3])/sqrt(2)
  Mux : Mux
  xd : Outport
  xq : Outport  Port=2
  wires:
  Mux/1 -> Fcn1/1, Fcn/1, Fcn2/1
  Fcn/1 -> xd/1
  Fcn1/1 -> xq/1
  xa/1 -> Mux/1
  xb/1 -> Mux/2
  xc/1 -> Mux/3
  theta/1 -> Mux/4

== system Lab4_6_StudentVersion/Droop Control/Freq Droop Modified/abc to dq1 ==
  xa : Inport
  xb : Inport  Port=2
  xc : Inport  Port=3
  theta : Inport  Port=4
  Fcn : Fcn  Expr=sqrt(2/3)*(u[1]*cos(u[4])+u[2]*cos(u[4]-2*pi/3)+u[3]*cos(u[4]-4*pi/3))
  Fcn1 : Fcn  Expr=sqrt(2/3)*(-u[1]*sin(u[4])-u[2]*sin(u[4]-2*pi/3)-u[3]*sin(u[4]-4*pi/3))
  Fcn2 : Fcn  Expr=sqrt(2/3)*(u[1]+u[2]+u[3])/sqrt(2)
  Mux : Mux
  xd : Outport
  xq : Outport  Port=2
  wires:
  theta/1 -> Mux/4
  xc/1 -> Mux/3
  xb/1 -> Mux/2
  xa/1 -> Mux/1
  Fcn1/1 -> xq/1
  Fcn/1 -> xd/1
  Mux/1 -> Fcn2/1, Fcn/1, Fcn1/1

== system Lab4_6_StudentVersion/Measurements/Subsystem/Subsystem2 ==
  V : Inport
  Abs1 : Abs  SaturateOnIntegerOverflow=off
  Constant5 : Constant  Value=1e-7
  Relational Operator : RelationalOperator  OutDataTypeStr=boolean  InputSameDT=off
  Switch : Switch  SaturateOnIntegerOverflow=off  InputSameDT=off
  out : Outport  VectorParamsAs1DForOutWhenUnconnected=off
  wires:
  Switch/1 -> out/1
  Constant5/1 -> Relational Operator/2, Switch/3
  Relational Operator/1 -> Switch/2
  V/1 -> Switch/1, Abs1/1
  Abs1/1 -> Relational Operator/1

== system Lab4_6_StudentVersion/Measurements/Subsystem2/Subsystem2 ==
  V : Inport
  Abs1 : Abs  SaturateOnIntegerOverflow=off
  Constant5 : Constant  Value=1e-7
  Relational Operator : RelationalOperator  OutDataTypeStr=boolean  InputSameDT=off
  Switch : Switch  SaturateOnIntegerOverflow=off  InputSameDT=off
  out : Outport  VectorParamsAs1DForOutWhenUnconnected=off
  wires:
  Abs1/1 -> Relational Operator/1
  V/1 -> Abs1/1, Switch/1
  Relational Operator/1 -> Switch/2
  Constant5/1 -> Switch/3, Relational Operator/2
  Switch/1 -> out/1
